simulink model "RLFactoryEnforceCrash2Opponents"  (R2020a)
settings: Solver=VariableStepAuto  StartTime=0.0  StopTime=10.0  RelTol=1e-3
undefined symbols (not defined in the file): BLOCKEDTIMER, EPS, getRandomSafeCoord, GoalRange, MAXVELOA, MAXVELOB, RLStartX, RLStartY, SAFETYDISTANCEA, SAFETYDISTANCEB, THRESHOLDA, THRESHOLDB, TSA, TSB, TSRL
libraries: rllib x1
(part 2 of 2)

== system RLFactoryEnforceCrash2Opponents/RLServiceAOpponent/RLServiceAOpponentController/RLServiceArrivedChecker/RLServiceEuclideanDistanceCalculator1 ==
  X : Inport
  Y : Inport  Port=2
  GoalX : Inport  Port=3
  GoalY : Inport  Port=4
  Square : Math  Operator=square  SaturateOnIntegerOverflow=on
  Square Root : Sqrt  SaturateOnIntegerOverflow=on
  Square1 : Math  Operator=square  SaturateOnIntegerOverflow=on
  Sum1 : Sum
  Sum3 : Sum  Inputs=+-
  Sum4 : Sum  Inputs=+-
  DistToGoal : Outport
  wires:
  GoalX/1 -> Sum3/2
  X/1 -> Sum3/1
  Sum1/1 -> Square Root/1
  Sum4/1 -> Square1/1
  Square/1 -> Sum1/1
  Y/1 -> Sum4/1
  Square Root/1 -> DistToGoal/1
  Square1/1 -> Sum1/2
  Sum3/1 -> Square/1
  GoalY/1 -> Sum4/2

== system RLFactoryEnforceCrash2Opponents/RLServiceAOpponent/RLServiceAOpponentController/RLServiceArrivedChecker/RLServiceEuclideanDistanceCalculator2 ==
  X : Inport
  Y : Inport  Port=2
  GoalX : Inport  Port=3
  GoalY : Inport  Port=4
  Square : Math  Operator=square  SaturateOnIntegerOverflow=on
  Square Root : Sqrt  SaturateOnIntegerOverflow=on
  Square1 : Math  Operator=square  SaturateOnIntegerOverflow=on
  Sum1 : Sum
  Sum3 : Sum  Inputs=+-
  Sum4 : Sum  Inputs=+-
  OppDistToGoal : Outport
  wires:
  GoalX/1 -> Sum3/2
  X/1 -> Sum3/1
  Sum1/1 -> Square Root/1
  Sum4/1 -> Square1/1
  Square/1 -> Sum1/1
  Y/1 -> Sum4/1
  Square Root/1 -> OppDistToGoal/1
  Square1/1 -> Sum1/2
  Sum3/1 -> Square/1
  GoalY/1 -> Sum4/2

== system RLFactoryEnforceCrash2Opponents/RLServiceBOpponent/RLServiceAOpponentController/RLServiceArrivedChecker/RLServiceEuclideanDistanceCalculator1 ==
  X : Inport
  Y : Inport  Port=2
  GoalX : Inport  Port=3
  GoalY : Inport  Port=4
  Square : Math  Operator=square  SaturateOnIntegerOverflow=on
  Square Root : Sqrt  SaturateOnIntegerOverflow=on
  Square1 : Math  Operator=square  SaturateOnIntegerOverflow=on
  Sum1 : Sum
  Sum3 : Sum  Inputs=+-
  Sum4 : Sum  Inputs=+-
  DistToGoal : Outport
  wires:
  GoalX/1 -> Sum3/2
  X/1 -> Sum3/1
  Sum1/1 -> Square Root/1
  Sum4/1 -> Square1/1
  Square/1 -> Sum1/1
  Y/1 -> Sum4/1
  Square Root/1 -> DistToGoal/1
  Square1/1 -> Sum1/2
  Sum3/1 -> Square/1
  GoalY/1 -> Sum4/2

== system RLFactoryEnforceCrash2Opponents/RLServiceBOpponent/RLServiceAOpponentController/RLServiceArrivedChecker/RLServiceEuclideanDistanceCalculator2 ==
  X : Inport
  Y : Inport  Port=2
  GoalX : Inport  Port=3
  GoalY : Inport  Port=4
  Square : Math  Operator=square  SaturateOnIntegerOverflow=on
  Square Root : Sqrt  SaturateOnIntegerOverflow=on
  Square1 : Math  Operator=square  SaturateOnIntegerOverflow=on
  Sum1 : Sum
  Sum3 : Sum  Inputs=+-
  Sum4 : Sum  Inputs=+-
  OppDistToGoal : Outport
  wires:
  GoalX/1 -> Sum3/2
  X/1 -> Sum3/1
  Sum1/1 -> Square Root/1
  Sum4/1 -> Square1/1
  Square/1 -> Sum1/1
  Y/1 -> Sum4/1
  Square Root/1 -> OppDistToGoal/1
  Square1/1 -> Sum1/2
  Sum3/1 -> Square/1
  GoalY/1 -> Sum4/2
